simulink model "test_PLC_Drive_Rev3"  (R2020b)
settings: Solver=VariableStepAuto  StartTime=0.0  StopTime=t_stop  RelTol=1e-3
values from neighbouring files (symbols this model uses):
  Controller_sampleTime = 0.001    [PLC_setup_Rev1_02Mar21.m]    (also in PLC_setup_Rev3.m; PLC_setup_Rev4.m)
  Droop_scaling = 0    [PLC_setup_Rev1_02Mar21.m]    (also in PLC_setup_Rev3.m; PLC_setup_Rev4.m)
  VFD_acceleration_model_factor = 0.27*mmul2    (= 0.27)    [PLC_setup_Rev3.m]    (also in PLC_setup_Rev4.m)
  VFD_Adapt_factor_lower_p1458 = 1    [PLC_setup_Rev1_02Mar21.m]    (also in PLC_setup_Rev3.m; PLC_setup_Rev4.m)
  VFD_Adapt_factor_upper_p1459 = 1    [PLC_setup_Rev1_02Mar21.m]    (also in PLC_setup_Rev3.m; PLC_setup_Rev4.m)
  VFD_Curr_limit_var_p0641 = 1    [PLC_setup_Rev1_02Mar21.m]    (also in PLC_setup_Rev3.m; PLC_setup_Rev4.m)
  VFD_Current_limit_p0640 = 430    [PLC_setup_Rev1_02Mar21.m]    (also in PLC_setup_Rev3.m; PLC_setup_Rev4.m)
  VFD_Id_setp_total_r1624 = 73    [PLC_setup_Rev1_02Mar21.m]    (also in PLC_setup_Rev3.m; PLC_setup_Rev4.m)
  VFD_Iq = 1    [PLC_setup_Rev1_02Mar21.m]    (also in PLC_setup_Rev3.m; PLC_setup_Rev4.m)
  VFD_Kp_n_basic_p1460 = 20.174    [PLC_setup_Rev1_02Mar21.m]    (also in PLC_setup_Rev3.m; PLC_setup_Rev4.m)
  VFD_M = inf    [PLC_setup_Rev1_02Mar21.m]    (also in PLC_setup_Rev3.m; PLC_setup_Rev4.m)
  VFD_M_accel_T_smooth_p1517 = 4    [PLC_setup_Rev1_02Mar21.m]    (also in PLC_setup_Rev3.m; PLC_setup_Rev4.m)
  VFD_M_lim_var_fixS_src_p1551 = 1    [PLC_setup_Rev1_02Mar21.m]    (also in PLC_setup_Rev3.m; PLC_setup_Rev4.m)
  VFD_M_max_lower_p1521 = -1345    [PLC_setup_Rev1_02Mar21.m]    (also in PLC_setup_Rev3.m; PLC_setup_Rev4.m)
  VFD_M_max_lower_scal_p1525 = 1    [PLC_setup_Rev1_02Mar21.m]    (also in PLC_setup_Rev3.m; PLC_setup_Rev4.m)
  VFD_M_max_up_mot_scal_p1524 = 1    [PLC_setup_Rev1_02Mar21.m]    (also in PLC_setup_Rev3.m; PLC_setup_Rev4.m)
  VFD_M_max_upper_p1520 = 1345    [PLC_setup_Rev1_02Mar21.m]    (also in PLC_setup_Rev3.m; PLC_setup_Rev4.m)
  VFD_n_act_T_smooth_p1442 = 4    [PLC_setup_Rev1_02Mar21.m]    (also in PLC_setup_Rev3.m; PLC_setup_Rev4.m)
  VFD_n_ctr_Kp_n_up_scal_p1461 = 1    [PLC_setup_Rev1_02Mar21.m]    (also in PLC_setup_Rev3.m; PLC_setup_Rev4.m)
  VFD_n_ctr_Tn_n_up_sca_p1463 = 1    [PLC_setup_Rev1_02Mar21.m]    (also in PLC_setup_Rev3.m; PLC_setup_Rev4.m)
  VFD_n_ctrl_adapt_Kp_lower_p1456 = 0    [PLC_setup_Rev1_02Mar21.m]    (also in PLC_setup_Rev3.m; PLC_setup_Rev4.m)
  VFD_n_ctrl_adapt_Kp_upper_p1457 = 0.1    [PLC_setup_Rev1_02Mar21.m]    (also in PLC_setup_Rev3.m; PLC_setup_Rev4.m)
  VFD_n_ctrl_Adpt_sig_Kp_p1455 = 0    [PLC_setup_Rev1_02Mar21.m]    (also in PLC_setup_Rev3.m; PLC_setup_Rev4.m)
  VFD_n_ctrl_Kp_scal_p1466 = 1    [PLC_setup_Rev1_02Mar21.m]    (also in PLC_setup_Rev3.m; PLC_setup_Rev4.m)
  VFD_n_ctrl_n_lower_p1464 = 0    [PLC_setup_Rev1_02Mar21.m]    (also in PLC_setup_Rev3.m; PLC_setup_Rev4.m)
  VFD_n_ctrl_n_upper_p1465 = 1680    [PLC_setup_Rev1_02Mar21.m]    (also in PLC_setup_Rev3.m; PLC_setup_Rev4.m)
  VFD_n_ctrl_Tn_n_lower_p1462 = 96    [PLC_setup_Rev1_02Mar21.m]    (also in PLC_setup_Rev3.m; PLC_setup_Rev4.m)
  VFD_n_limit_neg_p1086 = -40000    [PLC_setup_Rev1_02Mar21.m]    (also in PLC_setup_Rev3.m; PLC_setup_Rev4.m)
  VFD_n_limit_pos_p1083 = 40000    [PLC_setup_Rev1_02Mar21.m]    (also in PLC_setup_Rev3.m; PLC_setup_Rev4.m)
  VFD_n_limit_setp_p1063 = 40000    [PLC_setup_Rev1_02Mar21.m]    (also in PLC_setup_Rev3.m; PLC_setup_Rev4.m)
  VFD_n_max_p1082 = 1680    [PLC_setup_Rev1_02Mar21.m]    (also in PLC_setup_Rev3.m; PLC_setup_Rev4.m)
  VFD_n_set_filt_1_T_p1416 = 0    [PLC_setup_Rev1_02Mar21.m]    (also in PLC_setup_Rev3.m; PLC_setup_Rev4.m)
  VFD_P_max_gen_p1531 = -375    [PLC_setup_Rev1_02Mar21.m]    (also in PLC_setup_Rev3.m; PLC_setup_Rev4.m)
  VFD_P_max_mot_p1530 = 125    [PLC_setup_Rev1_02Mar21.m]    (also in PLC_setup_Rev3.m; PLC_setup_Rev4.m)
  VFD_PU_I_outp_max_r0289 = 452    [PLC_setup_Rev1_02Mar21.m]    (also in PLC_setup_Rev3.m; PLC_setup_Rev4.m)
  VFD_RFG_ramp_down_time_p1121 = 0.7    [PLC_setup_Rev1_02Mar21.m]    (also in PLC_setup_Rev3.m; PLC_setup_Rev4.m)
  VFD_RFG_ramp_up_time_p1120 = 0.7    [PLC_setup_Rev1_02Mar21.m]    (also in PLC_setup_Rev3.m; PLC_setup_Rev4.m)
  VFD_RFG_t_RD_scal_p1139 = 1    [PLC_setup_Rev1_02Mar21.m]    (also in PLC_setup_Rev3.m; PLC_setup_Rev4.m)
  VFD_RFG_t_RU_scal_p1138 = 1    [PLC_setup_Rev1_02Mar21.m]    (also in PLC_setup_Rev3.m; PLC_setup_Rev4.m)
undefined symbols (not defined in the file or in its folder): DiscIntNeverNeededParam, filt_enc_den, filt_enc_num, filt_NUM, Kp_mul, tau_m, Tn_mul, Tsf
libraries: simulink x49, simulink_extras x1
(part 1 of 2)
settings Model: Creator=Pawel  LastModifiedBy=Pawel

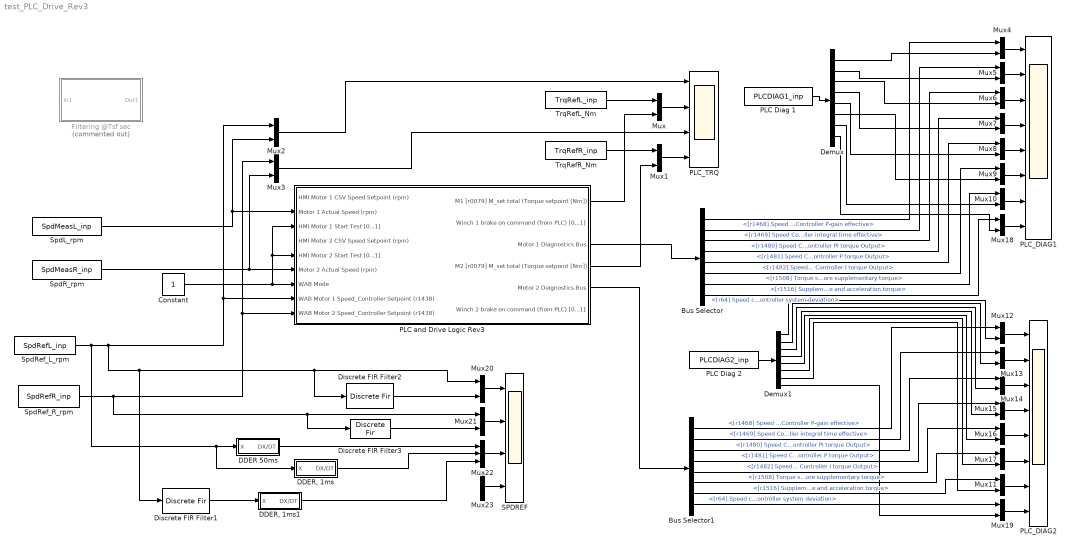
== system test_PLC_Drive_Rev3 ==
  Bus Selector : BusSelector  OutputSignals=signal1.[r1468] Speed Controller P-gain effective,signal1.[r1469] Speed Controller integral time effective,signal1.[r1480] Speed Controller PI torque Output,signal1.[r1481] Speed Controller P torque Output,signal1.[r1482] Speed Controller I torque Output,signal1.[r1508] Torque setpoint before supplementary torque,signal1.[r1516] Supplementary torque and acceleration torque,signal1.[r64] Speed controller system deviation
  Bus Selector1 : BusSelector  OutputSignals=signal1.[r1468] Speed Controller P-gain effective,signal1.[r1469] Speed Controller integral time effective,signal1.[r1480] Speed Controller PI torque Output,signal1.[r1481] Speed Controller P torque Output,signal1.[r1482] Speed Controller I torque Output,signal1.[r1508] Torque setpoint before supplementary torque,signal1.[r1516] Supplementary torque and acceleration torque,signal1.[r64] Speed controller system deviation
  Constant : Constant
  DDER 50ms : Subsystem  TreatAsAtomicUnit=on  SystemSampleTime=0.05
  "DDER, 1ms" : Subsystem  TreatAsAtomicUnit=on  SystemSampleTime=0.001
  "DDER, 1ms1" : Subsystem  TreatAsAtomicUnit=on  SystemSampleTime=0.001
  Demux : Demux  Outputs=8
  Demux1 : Demux  Outputs=8
  Discrete FIR Filter1 : DiscreteFir  Coefficients=filt_NUM  SampleTime=Controller_sampleTime
  Discrete FIR Filter2 : DiscreteFir  Coefficients=filt_NUM  SampleTime=Controller_sampleTime
  Discrete FIR Filter3 : DiscreteFir  Coefficients=filt_NUM  SampleTime=Controller_sampleTime
  Filtering @Tsf sec : Subsystem  Commented=on  TreatAsAtomicUnit=on  SystemSampleTime=Tsf
  Mux{,1..21} (22 alike) : Mux  Inputs=2
  Mux22 : Mux  Inputs=3
  Mux23 : Mux  Inputs=3
  PLC Diag 1 : FromWorkspace  VariableName=PLCDIAG1_inp  OutputAfterFinalValue=Holding final value
  PLC Diag 2 : FromWorkspace  VariableName=PLCDIAG2_inp  OutputAfterFinalValue=Holding final value
  PLC and Drive Logic Rev3 : Subsystem  AncestorBlock=Control_Library_Rev3/PLC and Drive Logic
  PLC_DIAG1 : Scope  NumInputPorts=8
  PLC_DIAG2 : Scope  NumInputPorts=8
  PLC_TRQ : Scope  NumInputPorts=4
  SPDREF : Scope  NumInputPorts=4
  SpdL_rpm : FromWorkspace  VariableName=SpdMeasL_inp  OutputAfterFinalValue=Holding final value
  SpdR_rpm : FromWorkspace  VariableName=SpdMeasR_inp  OutputAfterFinalValue=Holding final value
  SpdRef_L_rpm : FromWorkspace  VariableName=SpdRefL_inp  OutputAfterFinalValue=Holding final value
  SpdRef_R_rpm : FromWorkspace  VariableName=SpdRefR_inp  OutputAfterFinalValue=Holding final value
  TrqRefL_Nm : FromWorkspace  VariableName=TrqRefL_inp  OutputAfterFinalValue=Holding final value
  TrqRefR_Nm : FromWorkspace  VariableName=TrqRefR_inp  OutputAfterFinalValue=Holding final value
  wires:
  Constant/1 -> PLC and Drive Logic Rev3/7(WAB Mode), PLC and Drive Logic Rev3/3(HMI Motor 1 Start Test [0...1]), PLC and Drive Logic Rev3/5(HMI Motor 2 Start Test [0...1])
  PLC and Drive Logic Rev3/1(M1 [r0079] M_set total (Torque setpoint [Nm])) -> Mux/2
  PLC and Drive Logic Rev3/4(M2 [r0079] M_set total (Torque setpoint [Nm])) -> Mux1/2
  Mux/1 -> PLC_TRQ/2
  Mux1/1 -> PLC_TRQ/4
  Mux2/1 -> PLC_TRQ/1
  Mux3/1 -> PLC_TRQ/3
  TrqRefL_Nm/1 -> Mux/1
  TrqRefR_Nm/1 -> Mux1/1
  PLC and Drive Logic Rev3/3(Motor 1 Diagnostics Bus) -> Bus Selector/1
  Mux4/1 -> PLC_DIAG1/1
  Mux6/1 -> PLC_DIAG1/3
  Mux5/1 -> PLC_DIAG1/2
  Mux7/1 -> PLC_DIAG1/4
  Mux9/1 -> PLC_DIAG1/6
  Mux8/1 -> PLC_DIAG1/5
  Mux10/1 -> PLC_DIAG1/7
  Bus Selector/1 -> Mux4/1  "<[r1468] Speed Controller P-gain effective>"
  Bus Selector/2 -> Mux5/1  "<[r1469] Speed Controller integral time effective>"
  Bus Selector/3 -> Mux6/1  "<[r1480] Speed Controller PI torque Output>"
  Bus Selector/4 -> Mux7/1  "<[r1481] Speed Controller P torque Output>"
  Bus Selector/5 -> Mux8/1  "<[r1482] Speed Controller I torque Output>"
  Bus Selector/6 -> Mux9/1  "<[r1508] Torque setpoint before supplementary torque>"
  Bus Selector/7 -> Mux10/1  "<[r1516] Supplementary torque and acceleration torque>"
  PLC and Drive Logic Rev3/5(Motor 2 Diagnostics Bus) -> Bus Selector1/1
  Bus Selector1/7 -> Mux11/1  "<[r1516] Supplementary torque and acceleration torque>"
  Bus Selector1/6 -> Mux17/1  "<[r1508] Torque setpoint before supplementary torque>"
  Bus Selector1/5 -> Mux16/1  "<[r1482] Speed Controller I torque Output>"
  Bus Selector1/4 -> Mux15/1  "<[r1481] Speed Controller P torque Output>"
  Bus Selector1/3 -> Mux14/1  "<[r1480] Speed Controller PI torque Output>"
  Bus Selector1/2 -> Mux13/1  "<[r1469] Speed Controller integral time effective>"
  Bus Selector1/1 -> Mux12/1  "<[r1468] Speed Controller P-gain effective>"
  Mux11/1 -> PLC_DIAG2/7
  Mux16/1 -> PLC_DIAG2/5
  Mux17/1 -> PLC_DIAG2/6
  Mux15/1 -> PLC_DIAG2/4
  Mux13/1 -> PLC_DIAG2/2
  Mux14/1 -> PLC_DIAG2/3
  Mux12/1 -> PLC_DIAG2/1
  SpdRef_R_rpm/1 -> PLC and Drive Logic Rev3/9(WAB Motor 2 Speed_Controller Setpoint (r1438)), Mux3/1, Discrete FIR Filter3/1, Mux21/1
  SpdRef_L_rpm/1 -> "DDER, 1ms"/1(X), DDER 50ms/1(X), PLC and Drive Logic Rev3/8(WAB Motor 1 Speed_Controller Setpoint (r1438)), Mux2/1, Discrete FIR Filter1/1, Discrete FIR Filter2/1, Mux20/1
  SpdR_rpm/1 -> PLC and Drive Logic Rev3/6(Motor 2 Actual Speed (rpm)), Mux3/2
  SpdL_rpm/1 -> PLC and Drive Logic Rev3/2(Motor 1 Actual Speed (rpm)), Mux2/2
  PLC Diag 1/1 -> Demux/1
  Demux/1 -> Mux4/2
  Demux/2 -> Mux5/2
  Demux/3 -> Mux6/2
  Demux/4 -> Mux7/2
  Demux/5 -> Mux8/2
  Demux/6 -> Mux9/2
  Demux/7 -> Mux10/2
  PLC Diag 2/1 -> Demux1/1
  Demux1/1 -> Mux12/2
  Demux1/2 -> Mux13/2
  Demux1/3 -> Mux14/2
  Demux1/4 -> Mux15/2
  Demux1/5 -> Mux16/2
  Demux1/6 -> Mux17/2
  Demux1/7 -> Mux11/2
  Mux18/1 -> PLC_DIAG1/8
  Mux19/1 -> PLC_DIAG2/8
  Bus Selector/8 -> Mux18/1  "<[r64] Speed controller system deviation>"
  Bus Selector1/8 -> Mux19/1  "<[r64] Speed controller system deviation>"
  Demux/8 -> Mux18/2
  Demux1/8 -> Mux19/2
  Mux20/1 -> SPDREF/1
  Mux21/1 -> SPDREF/2
  Mux23/1 -> SPDREF/4
  Mux22/1 -> SPDREF/3
  DDER 50ms/1(DX/DT) -> Mux22/1
  "DDER, 1ms"/1(DX/DT) -> Mux22/2
  "DDER, 1ms1"/1(DX/DT) -> Mux22/3
  Discrete FIR Filter1/1 -> "DDER, 1ms1"/1(X)
  Discrete FIR Filter2/1 -> Mux20/2
  Discrete FIR Filter3/1 -> Mux21/2

== system test_PLC_Drive_Rev3/DDER 50ms ==
  X : Inport
  Discrete Derivative : simulink/Discrete/Discrete Derivative  gainval=1.0  ICPrevScaledInput=0.0  OutMin=[]  OutMax=[]  OutDataType=fixdt(1, 16)  OutScaling=2^-10  DoSatur=off
  DX/DT : Outport
  wires:
  Discrete Derivative/1 -> DX/DT/1
  X/1 -> Discrete Derivative/1

== system test_PLC_Drive_Rev3/DDER, 1ms ==
  X : Inport
  Discrete Derivative : simulink/Discrete/Discrete Derivative  gainval=1.0  ICPrevScaledInput=0.0  OutMin=[]  OutMax=[]  OutDataType=fixdt(1, 16)  OutScaling=2^-10  DoSatur=off
  DX/DT : Outport
  wires:
  X/1 -> Discrete Derivative/1
  Discrete Derivative/1 -> DX/DT/1

== system test_PLC_Drive_Rev3/DDER, 1ms1 ==
  X : Inport
  Discrete Derivative : simulink/Discrete/Discrete Derivative  gainval=1.0  ICPrevScaledInput=0.0  OutMin=[]  OutMax=[]  OutDataType=fixdt(1, 16)  OutScaling=2^-10  DoSatur=off
  DX/DT : Outport
  wires:
  Discrete Derivative/1 -> DX/DT/1
  X/1 -> Discrete Derivative/1

== system test_PLC_Drive_Rev3/Filtering @Tsf sec ==
  In1 : Inport
  Filter2 : simulink_extras/Additional Discrete/Discrete Transfer Fcn (with initial outputs)  N=filt_enc_num  D=filt_enc_den  U0=qA_0  Y0=qA_0  TS=-1
      settings: SourceProductBaseCode=SL
  Out1 : Outport

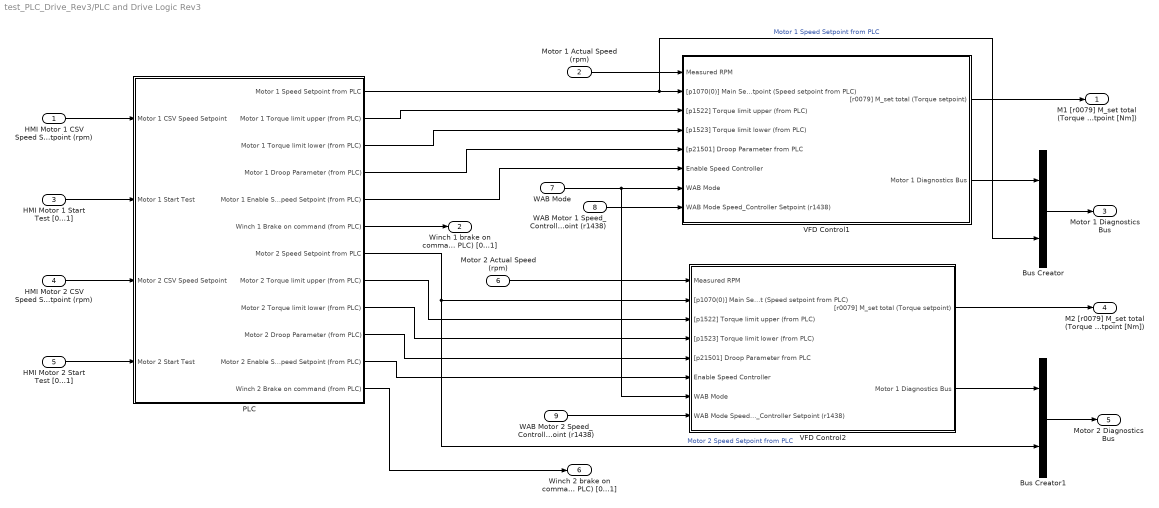
== system test_PLC_Drive_Rev3/PLC and Drive Logic Rev3 ==
  HMI Motor 1 CSV Speed Setpoint (rpm) : Inport
  Motor 1 Actual Speed (rpm) : Inport  Port=2
  HMI Motor 1 Start Test [0...1] : Inport  Port=3
  HMI Motor 2 CSV Speed Setpoint (rpm) : Inport  Port=4
  HMI Motor 2 Start Test [0...1] : Inport  Port=5
  Motor 2 Actual Speed (rpm) : Inport  Port=6
  WAB Mode : Inport  Port=7
  WAB Motor 1 Speed_Controller Setpoint (r1438) : Inport  Port=8
  WAB Motor 2 Speed_Controller Setpoint (r1438) : Inport  Port=9
  Bus Creator : BusCreator  Inputs=2
  Bus Creator1 : BusCreator  Inputs=2
  PLC : Subsystem  TreatAsAtomicUnit=on  SystemSampleTime=Controller_sampleTime
  VFD Control1 : Subsystem  AncestorBlock=Control_Library_Rev3/VFD Control  TreatAsAtomicUnit=on  SystemSampleTime=Controller_sampleTime
  VFD Control2 : Subsystem  AncestorBlock=Control_Library_Rev3/VFD Control  TreatAsAtomicUnit=on  SystemSampleTime=Controller_sampleTime
  M1 [r0079] M_set total (Torque setpoint [Nm]) : Outport
  Winch 1 brake on command (from PLC) [0...1] : Outport  Port=2
  Motor 1 Diagnostics Bus : Outport  Port=3
  M2 [r0079] M_set total (Torque setpoint [Nm]) : Outport  Port=4
  Motor 2 Diagnostics Bus : Outport  Port=5
  Winch 2 brake on command (from PLC) [0...1] : Outport  Port=6
  wires:
  PLC/3(Motor 1 Torque limit lower (from PLC)) -> VFD Control1/4("[p1523] Torque limit lower (from PLC)")
  Motor 1 Actual Speed (rpm)/1 -> VFD Control1/1(Measured RPM)
  PLC/2(Motor 1 Torque limit upper (from PLC)) -> VFD Control1/3("[p1522] Torque limit upper (from PLC)")
  PLC/1(Motor 1 Speed Setpoint from PLC) -> VFD Control1/2("[p1070(0)] Main Setpoint (Speed setpoint from PLC)"), Bus Creator/2  "Motor 1 Speed Setpoint from PLC"
  HMI Motor 1 Start Test [0...1]/1 -> PLC/2(Motor 1 Start Test)
  VFD Control1/1("[r0079] M_set total (Torque setpoint)") -> M1 [r0079] M_set total (Torque setpoint [Nm])/1
  HMI Motor 1 CSV Speed Setpoint (rpm)/1 -> PLC/1(Motor 1 CSV Speed Setpoint)
  PLC/4(Motor 1 Droop Parameter (from PLC)) -> VFD Control1/5("[p21501] Droop Parameter from PLC")
  PLC/5(Motor 1 Enable Speed Setpoint (from PLC)) -> VFD Control1/6(Enable Speed Controller)
  VFD Control1/2(Motor 1 Diagnostics Bus) -> Bus Creator/1
  Bus Creator/1 -> Motor 1 Diagnostics Bus/1
  Bus Creator1/1 -> Motor 2 Diagnostics Bus/1
  VFD Control2/2(Motor 1 Diagnostics Bus) -> Bus Creator1/1
  VFD Control2/1("[r0079] M_set total (Torque setpoint)") -> M2 [r0079] M_set total (Torque setpoint [Nm])/1
  PLC/6(Winch 1 Brake on command (from PLC)) -> Winch 1 brake on command (from PLC) [0...1]/1
  HMI Motor 2 CSV Speed Setpoint (rpm)/1 -> PLC/3(Motor 2 CSV Speed Setpoint)
  HMI Motor 2 Start Test [0...1]/1 -> PLC/4(Motor 2 Start Test)
  Motor 2 Actual Speed (rpm)/1 -> VFD Control2/1(Measured RPM)
  PLC/7(Motor 2 Speed Setpoint from PLC) -> Bus Creator1/2, VFD Control2/2("[p1070(0)] Main Setpoint (Speed setpoint from PLC)")  "Motor 2 Speed Setpoint from PLC"
  PLC/8(Motor 2 Torque limit upper (from PLC)) -> VFD Control2/3("[p1522] Torque limit upper (from PLC)")
  PLC/9(Motor 2 Torque limit lower (from PLC)) -> VFD Control2/4("[p1523] Torque limit lower (from PLC)")
  PLC/10(Motor 2 Droop Parameter (from PLC)) -> VFD Control2/5("[p21501] Droop Parameter from PLC")
  PLC/11(Motor 2 Enable Speed Setpoint (from PLC)) -> VFD Control2/6(Enable Speed Controller)
  PLC/12(Winch 2 Brake on command (from PLC)) -> Winch 2 brake on command (from PLC) [0...1]/1
  WAB Motor 1 Speed_Controller Setpoint (r1438)/1 -> VFD Control1/8(WAB Mode Speed_Controller Setpoint (r1438))
  WAB Mode/1 -> VFD Control2/7(WAB Mode), VFD Control1/7(WAB Mode)
  WAB Motor 2 Speed_Controller Setpoint (r1438)/1 -> VFD Control2/8(WAB Mode Speed_Controller Setpoint (r1438))

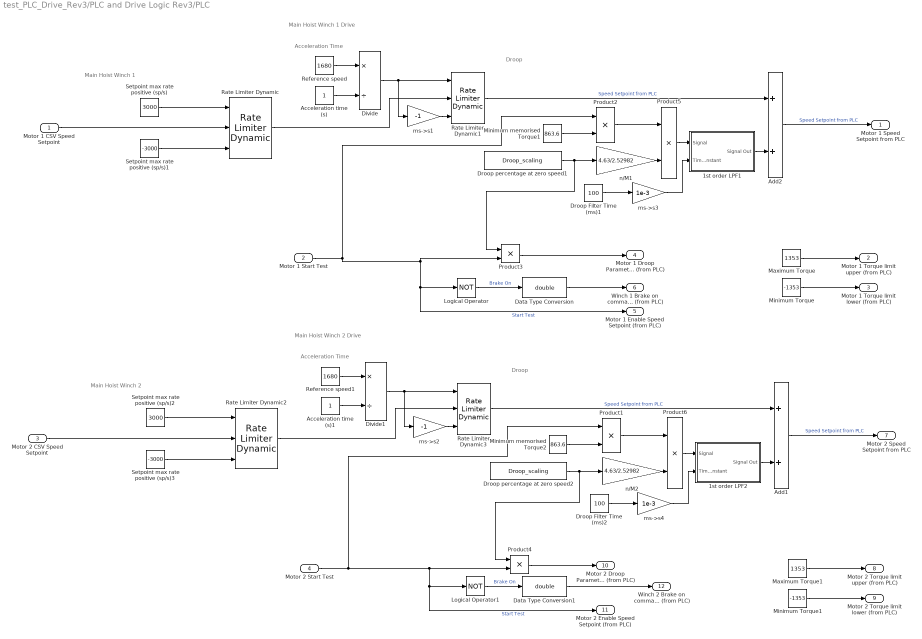
== system test_PLC_Drive_Rev3/PLC and Drive Logic Rev3/PLC ==
  note: Main Hoist Winch 1 Drive
  note: Acceleration Time
  note: Droop
  note: Main Hoist Winch 1
  note: Main Hoist Winch 2 Drive
  note: Acceleration Time
  note: Droop
  note: Main Hoist Winch 2
  Motor 1 CSV Speed Setpoint : Inport
  Motor 1 Start Test : Inport  Port=2
  Motor 2 CSV Speed Setpoint : Inport  Port=3
  Motor 2 Start Test : Inport  Port=4
  1st order LPF1 : Subsystem  mask{time_constant=0.1, Yo=0}
      mask prompts: time_constant "Time Constant (s)"; Yo "Initial Condition"
  1st order LPF2 : Subsystem  mask{time_constant=0.1, Yo=0}
      mask prompts: time_constant "Time Constant (s)"; Yo "Initial Condition"
  Acceleration time (s) : Constant
  Acceleration time (s)1 : Constant
  Add1 : Sum
  Add2 : Sum
  Data Type Conversion : DataTypeConversion  OutDataTypeStr=double
  Data Type Conversion1 : DataTypeConversion  OutDataTypeStr=double
  Divide : Product  Inputs=*/
  Divide1 : Product  Inputs=*/
  Droop Filter Time (ms)1 : Constant  Value=100
  Droop Filter Time (ms)2 : Constant  Value=100
  Droop percentage at zero speed1 : Constant  Value=Droop_scaling
  Droop percentage at zero speed2 : Constant  Value=Droop_scaling
  Logical Operator : Logic  Operator=NOT  AllPortsSameDT=off  OutDataTypeStr=boolean
  Logical Operator1 : Logic  Operator=NOT  AllPortsSameDT=off  OutDataTypeStr=boolean
  Maximum Torque : Constant  Value=1353
  Maximum Torque1 : Constant  Value=1353
  Minimum Torque : Constant  Value=-1353
  Minimum Torque1 : Constant  Value=-1353
  Minimum memorised Torque1 : Constant  Value=863.6
  Minimum memorised Torque2 : Constant  Value=863.6
  Product{1..2,5..6} (4 alike) : Product  Inputs=**
  Product3 : Product
  Product4 : Product
  Rate Limiter Dynamic{,1..3} (4 alike) : simulink/Discontinuities/Rate Limiter Dynamic
  Reference speed : Constant  Value=1680
  Reference speed1 : Constant  Value=1680
  Setpoint max rate positive (sp/s) : Constant  Value=3000
  Setpoint max rate positive (sp/s)1 : Constant  Value=-3000
  Setpoint max rate positive (sp/s)2 : Constant  Value=3000
  Setpoint max rate positive (sp/s)3 : Constant  Value=-3000
  ms->s1 : Gain  Gain=-1
  ms->s2 : Gain  Gain=-1
  ms->s3 : Gain  Gain=1e-3
  ms->s4 : Gain  Gain=1e-3
  n/M1 : Gain  Gain=4.63/2.52982
  n/M2 : Gain  Gain=4.63/2.52982
  Motor 1 Speed Setpoint from PLC : Outport
  Motor 1 Torque limit upper (from PLC) : Outport  Port=2
  Motor 1 Torque limit lower (from PLC) : Outport  Port=3
  Motor 1 Droop Parameter (from PLC) : Outport  Port=4
  Motor 1 Enable Speed Setpoint (from PLC) : Outport  Port=5
  Winch 1 Brake on command (from PLC) : Outport  Port=6
  Motor 2 Speed Setpoint from PLC : Outport  Port=7
  Motor 2 Torque limit upper (from PLC) : Outport  Port=8
  Motor 2 Torque limit lower (from PLC) : Outport  Port=9
  Motor 2 Droop Parameter (from PLC) : Outport  Port=10
  Motor 2 Enable Speed Setpoint (from PLC) : Outport  Port=11
  Winch 2 Brake on command (from PLC) : Outport  Port=12
  wires:
  Product2/1 -> Product5/1
  n/M1/1 -> Product5/2
  ms->s1/1 -> Rate Limiter Dynamic1/3
  ms->s3/1 -> 1st order LPF1/2(Time Constant)
  Divide/1 -> ms->s1/1, Rate Limiter Dynamic1/1
  Setpoint max rate positive (sp/s)/1 -> Rate Limiter Dynamic/1
  Setpoint max rate positive (sp/s)1/1 -> Rate Limiter Dynamic/3
  Product5/1 -> 1st order LPF1/1(Signal)
  Droop Filter Time (ms)1/1 -> ms->s3/1
  1st order LPF1/1(Signal Out) -> Add2/2
  Droop percentage at zero speed1/1 -> Product3/1, n/M1/1
  Rate Limiter Dynamic/1 -> Rate Limiter Dynamic1/2
  Minimum memorised Torque1/1 -> Product2/2
  Reference speed/1 -> Divide/1
  Acceleration time (s)/1 -> Divide/2
  Add2/1 -> Motor 1 Speed Setpoint from PLC/1  "Speed Setpoint from PLC"
  Maximum Torque/1 -> Motor 1 Torque limit upper (from PLC)/1
  Minimum Torque/1 -> Motor 1 Torque limit lower (from PLC)/1
  Rate Limiter Dynamic1/1 -> Add2/1  "Speed Setpoint from PLC"
  Motor 1 Start Test/1 -> Motor 1 Enable Speed Setpoint (from PLC)/1, Logical Operator/1, Product3/2, Product2/1  "Start Test"
  Product3/1 -> Motor 1 Droop Parameter (from PLC)/1
  Logical Operator/1 -> Data Type Conversion/1  "Brake On"
  Data Type Conversion/1 -> Winch 1 Brake on command (from PLC)/1
  Motor 1 CSV Speed Setpoint/1 -> Rate Limiter Dynamic/2
  Motor 2 CSV Speed Setpoint/1 -> Rate Limiter Dynamic2/2
  Data Type Conversion1/1 -> Winch 2 Brake on command (from PLC)/1
  Logical Operator1/1 -> Data Type Conversion1/1  "Brake On"
  Product4/1 -> Motor 2 Droop Parameter (from PLC)/1
  Motor 2 Start Test/1 -> Product1/1, Motor 2 Enable Speed Setpoint (from PLC)/1, Logical Operator1/1, Product4/2  "Start Test"
  Rate Limiter Dynamic3/1 -> Add1/1  "Speed Setpoint from PLC"
  Minimum Torque1/1 -> Motor 2 Torque limit lower (from PLC)/1
  Maximum Torque1/1 -> Motor 2 Torque limit upper (from PLC)/1
  Add1/1 -> Motor 2 Speed Setpoint from PLC/1  "Speed Setpoint from PLC"
  Acceleration time (s)1/1 -> Divide1/2
  Reference speed1/1 -> Divide1/1
  Minimum memorised Torque2/1 -> Product1/2
  Rate Limiter Dynamic2/1 -> Rate Limiter Dynamic3/2
  Droop percentage at zero speed2/1 -> n/M2/1, Product4/1
  1st order LPF2/1(Signal Out) -> Add1/2
  Droop Filter Time (ms)2/1 -> ms->s4/1
  Product6/1 -> 1st order LPF2/1(Signal)
  Setpoint max rate positive (sp/s)3/1 -> Rate Limiter Dynamic2/3
  Setpoint max rate positive (sp/s)2/1 -> Rate Limiter Dynamic2/1
  Divide1/1 -> Rate Limiter Dynamic3/1, ms->s2/1
  ms->s4/1 -> 1st order LPF2/2(Time Constant)
  ms->s2/1 -> Rate Limiter Dynamic3/3
  n/M2/1 -> Product6/2
  Product1/1 -> Product6/1

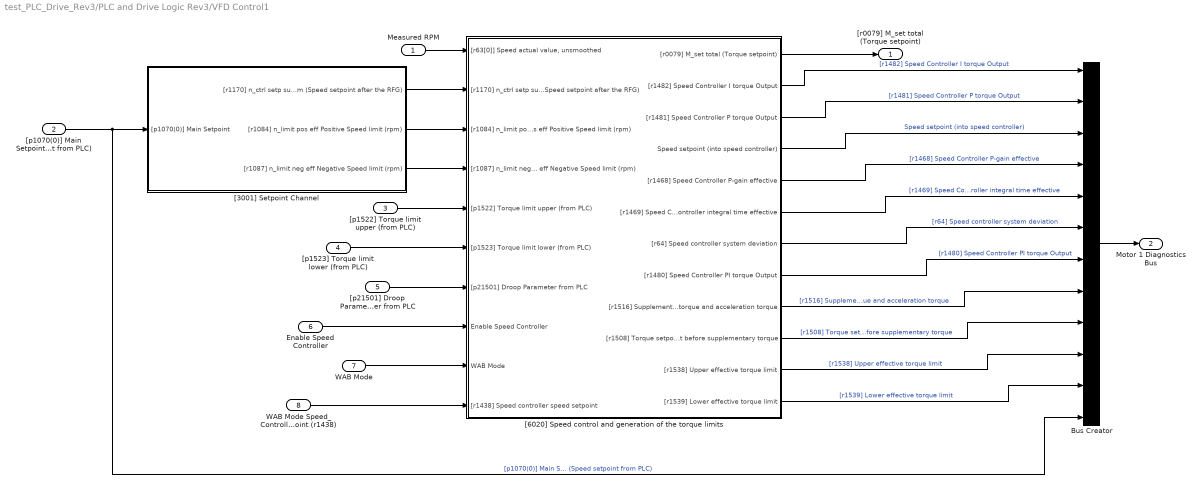
== system test_PLC_Drive_Rev3/PLC and Drive Logic Rev3/VFD Control1 ==
  Measured RPM : Inport
  "[p1070(0)] Main Setpoint (Speed setpoint from PLC)" : Inport  Port=2
  "[p1522] Torque limit upper (from PLC)" : Inport  Port=3
  "[p1523] Torque limit lower (from PLC)" : Inport  Port=4
  "[p21501] Droop Parameter from PLC" : Inport  Port=5
  Enable Speed Controller : Inport  Port=6
  WAB Mode : Inport  Port=7
  WAB Mode Speed_Controller Setpoint (r1438) : Inport  Port=8
  Bus Creator : BusCreator  Inputs=12
  "[3001] Setpoint Channel " : Subsystem
  "[6020] Speed control and generation of the torque limits " : Subsystem
  "[r0079] M_set total (Torque setpoint)" : Outport  VectorParamsAs1DForOutWhenUnconnected=off
  Motor 1 Diagnostics Bus : Outport  Port=2
  wires:
  "[6020] Speed control and generation of the torque limits "/12("[r1539] Lower effective torque limit") -> Bus Creator/11  "[r1539] Lower effective torque limit"
  "[6020] Speed control and generation of the torque limits "/11("[r1538] Upper effective torque limit") -> Bus Creator/10  "[r1538] Upper effective torque limit"
  "[6020] Speed control and generation of the torque limits "/10("[r1508] Torque setpoint before supplementary torque") -> Bus Creator/9  "[r1508] Torque setpoint before supplementary torque"
  "[6020] Speed control and generation of the torque limits "/9("[r1516] Supplementary torque and acceleration torque ") -> Bus Creator/8  "[r1516] Supplementary torque and acceleration torque"
  "[6020] Speed control and generation of the torque limits "/8("[r1480] Speed Controller PI torque Output") -> Bus Creator/7  "[r1480] Speed Controller PI torque Output"
  "[6020] Speed control and generation of the torque limits "/7("[r64] Speed controller system deviation") -> Bus Creator/6  "[r64] Speed controller system deviation"
  "[6020] Speed control and generation of the torque limits "/6("[r1469] Speed Controller integral time effective") -> Bus Creator/5  "[r1469] Speed Controller integral time effective"
  "[6020] Speed control and generation of the torque limits "/5("[r1468] Speed Controller P-gain effective") -> Bus Creator/4  "[r1468] Speed Controller P-gain effective"
  Bus Creator/1 -> Motor 1 Diagnostics Bus/1
  WAB Mode Speed_Controller Setpoint (r1438)/1 -> "[6020] Speed control and generation of the torque limits "/10("[r1438] Speed controller speed setpoint")
  WAB Mode/1 -> "[6020] Speed control and generation of the torque limits "/9(WAB Mode)
  "[6020] Speed control and generation of the torque limits "/2("[r1482] Speed Controller I torque Output") -> Bus Creator/1  "[r1482] Speed Controller I torque Output"
  "[6020] Speed control and generation of the torque limits "/3("[r1481] Speed Controller P torque Output") -> Bus Creator/2  "[r1481] Speed Controller P torque Output"
  Measured RPM/1 -> "[6020] Speed control and generation of the torque limits "/1("[r63[0]] Speed actual value, unsmoothed")
  "[p1070(0)] Main Setpoint (Speed setpoint from PLC)"/1 -> Bus Creator/12, "[3001] Setpoint Channel "/1("[p1070(0)] Main Setpoint")  "[p1070(0)] Main Setpoint (Speed setpoint from PLC)"
  "[3001] Setpoint Channel "/1("[r1170] n_ctrl setp sum (Speed setpoint after the RFG)") -> "[6020] Speed control and generation of the torque limits "/2("[r1170] n_ctrl setp sum (Speed setpoint after the RFG)")
  "[3001] Setpoint Channel "/2("[r1084] n_limit pos eff Positive Speed limit (rpm)") -> "[6020] Speed control and generation of the torque limits "/3("[r1084] n_limit pos eff Positive Speed limit (rpm)")
  "[3001] Setpoint Channel "/3("[r1087] n_limit neg eff Negative Speed limit (rpm)") -> "[6020] Speed control and generation of the torque limits "/4("[r1087] n_limit neg eff Negative Speed limit (rpm)")
  "[6020] Speed control and generation of the torque limits "/4(Speed setpoint (into speed controller)) -> Bus Creator/3  "Speed setpoint (into speed controller)"
  "[6020] Speed control and generation of the torque limits "/1("[r0079] M_set total (Torque setpoint)") -> "[r0079] M_set total (Torque setpoint)"/1
  "[p1523] Torque limit lower (from PLC)"/1 -> "[6020] Speed control and generation of the torque limits "/6("[p1523] Torque limit lower (from PLC)")
  "[p1522] Torque limit upper (from PLC)"/1 -> "[6020] Speed control and generation of the torque limits "/5("[p1522] Torque limit upper (from PLC)")
  "[p21501] Droop Parameter from PLC"/1 -> "[6020] Speed control and generation of the torque limits "/7("[p21501] Droop Parameter from PLC")
  Enable Speed Controller/1 -> "[6020] Speed control and generation of the torque limits "/8(Enable Speed Controller)

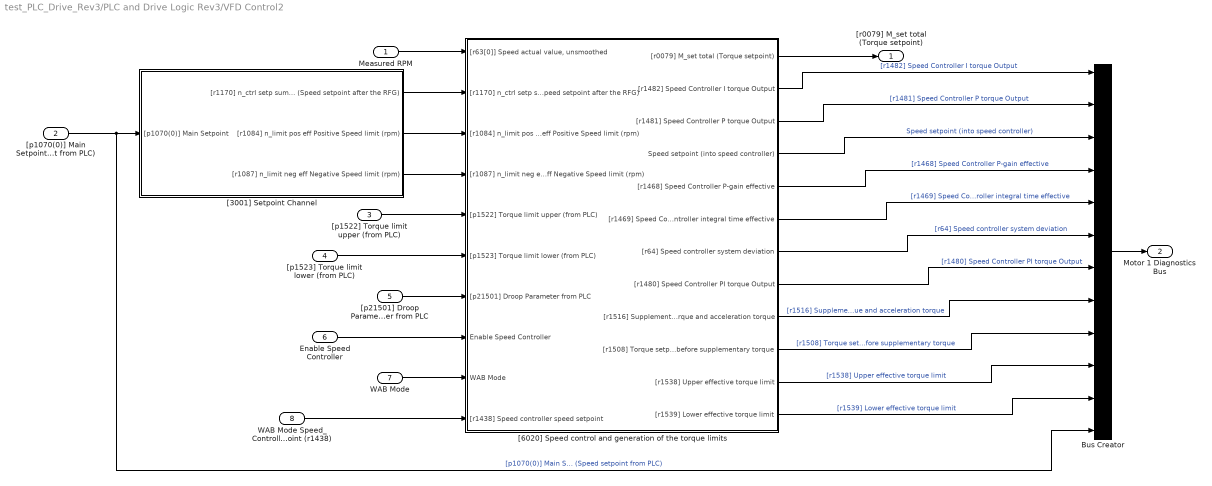
== system test_PLC_Drive_Rev3/PLC and Drive Logic Rev3/VFD Control2 ==
  Measured RPM : Inport
  "[p1070(0)] Main Setpoint (Speed setpoint from PLC)" : Inport  Port=2
  "[p1522] Torque limit upper (from PLC)" : Inport  Port=3
  "[p1523] Torque limit lower (from PLC)" : Inport  Port=4
  "[p21501] Droop Parameter from PLC" : Inport  Port=5
  Enable Speed Controller : Inport  Port=6
  WAB Mode : Inport  Port=7
  WAB Mode Speed_Controller Setpoint (r1438) : Inport  Port=8
  Bus Creator : BusCreator  Inputs=12
  "[3001] Setpoint Channel " : Subsystem
  "[6020] Speed control and generation of the torque limits " : Subsystem
  "[r0079] M_set total (Torque setpoint)" : Outport  VectorParamsAs1DForOutWhenUnconnected=off
  Motor 1 Diagnostics Bus : Outport  Port=2
  wires:
  "[6020] Speed control and generation of the torque limits "/12("[r1539] Lower effective torque limit") -> Bus Creator/11  "[r1539] Lower effective torque limit"
  "[6020] Speed control and generation of the torque limits "/11("[r1538] Upper effective torque limit") -> Bus Creator/10  "[r1538] Upper effective torque limit"
  "[6020] Speed control and generation of the torque limits "/10("[r1508] Torque setpoint before supplementary torque") -> Bus Creator/9  "[r1508] Torque setpoint before supplementary torque"
  "[6020] Speed control and generation of the torque limits "/9("[r1516] Supplementary torque and acceleration torque ") -> Bus Creator/8  "[r1516] Supplementary torque and acceleration torque"
  "[6020] Speed control and generation of the torque limits "/8("[r1480] Speed Controller PI torque Output") -> Bus Creator/7  "[r1480] Speed Controller PI torque Output"
  "[6020] Speed control and generation of the torque limits "/7("[r64] Speed controller system deviation") -> Bus Creator/6  "[r64] Speed controller system deviation"
  "[6020] Speed control and generation of the torque limits "/6("[r1469] Speed Controller integral time effective") -> Bus Creator/5  "[r1469] Speed Controller integral time effective"
  "[6020] Speed control and generation of the torque limits "/5("[r1468] Speed Controller P-gain effective") -> Bus Creator/4  "[r1468] Speed Controller P-gain effective"
  Bus Creator/1 -> Motor 1 Diagnostics Bus/1
  WAB Mode Speed_Controller Setpoint (r1438)/1 -> "[6020] Speed control and generation of the torque limits "/10("[r1438] Speed controller speed setpoint")
  WAB Mode/1 -> "[6020] Speed control and generation of the torque limits "/9(WAB Mode)
  "[6020] Speed control and generation of the torque limits "/2("[r1482] Speed Controller I torque Output") -> Bus Creator/1  "[r1482] Speed Controller I torque Output"
  "[6020] Speed control and generation of the torque limits "/3("[r1481] Speed Controller P torque Output") -> Bus Creator/2  "[r1481] Speed Controller P torque Output"
  Measured RPM/1 -> "[6020] Speed control and generation of the torque limits "/1("[r63[0]] Speed actual value, unsmoothed")
  "[p1070(0)] Main Setpoint (Speed setpoint from PLC)"/1 -> Bus Creator/12, "[3001] Setpoint Channel "/1("[p1070(0)] Main Setpoint")  "[p1070(0)] Main Setpoint (Speed setpoint from PLC)"
  "[3001] Setpoint Channel "/1("[r1170] n_ctrl setp sum (Speed setpoint after the RFG)") -> "[6020] Speed control and generation of the torque limits "/2("[r1170] n_ctrl setp sum (Speed setpoint after the RFG)")
  "[3001] Setpoint Channel "/2("[r1084] n_limit pos eff Positive Speed limit (rpm)") -> "[6020] Speed control and generation of the torque limits "/3("[r1084] n_limit pos eff Positive Speed limit (rpm)")
  "[3001] Setpoint Channel "/3("[r1087] n_limit neg eff Negative Speed limit (rpm)") -> "[6020] Speed control and generation of the torque limits "/4("[r1087] n_limit neg eff Negative Speed limit (rpm)")
  "[6020] Speed control and generation of the torque limits "/4(Speed setpoint (into speed controller)) -> Bus Creator/3  "Speed setpoint (into speed controller)"
  "[6020] Speed control and generation of the torque limits "/1("[r0079] M_set total (Torque setpoint)") -> "[r0079] M_set total (Torque setpoint)"/1
  "[p1523] Torque limit lower (from PLC)"/1 -> "[6020] Speed control and generation of the torque limits "/6("[p1523] Torque limit lower (from PLC)")
  "[p1522] Torque limit upper (from PLC)"/1 -> "[6020] Speed control and generation of the torque limits "/5("[p1522] Torque limit upper (from PLC)")
  "[p21501] Droop Parameter from PLC"/1 -> "[6020] Speed control and generation of the torque limits "/7("[p21501] Droop Parameter from PLC")
  Enable Speed Controller/1 -> "[6020] Speed control and generation of the torque limits "/8(Enable Speed Controller)

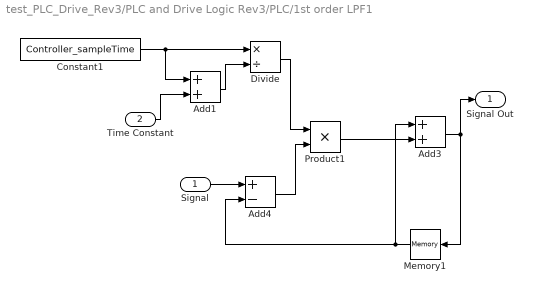
== system test_PLC_Drive_Rev3/PLC and Drive Logic Rev3/PLC/1st order LPF1 ==
  Signal : Inport
  Time Constant : Inport  Port=2
  Add1 : Sum
  Add3 : Sum
  Add4 : Sum  Inputs=+-
  Constant1 : Constant  Value=Controller_sampleTime
  Divide : Product  Inputs=*/
  Memory1 : Memory  InitialCondition=Yo  InheritSampleTime=on
  Product1 : Product  RndMeth=Zero
  Signal Out : Outport  VectorParamsAs1DForOutWhenUnconnected=off
  wires:
  Add1/1 -> Divide/2
  Divide/1 -> Product1/1
  Add3/1 -> Memory1/1, Signal Out/1
  Product1/1 -> Add3/2
  Memory1/1 -> Add4/2, Add3/1
  Add4/1 -> Product1/2
  Time Constant/1 -> Add1/2
  Constant1/1 -> Add1/1, Divide/1
  Signal/1 -> Add4/1

== system test_PLC_Drive_Rev3/PLC and Drive Logic Rev3/PLC/1st order LPF2 ==
  Signal : Inport
  Time Constant : Inport  Port=2
  Add1 : Sum
  Add3 : Sum
  Add4 : Sum  Inputs=+-
  Constant1 : Constant  Value=Controller_sampleTime
  Divide : Product  Inputs=*/
  Memory1 : Memory  InitialCondition=Yo  InheritSampleTime=on
  Product1 : Product  RndMeth=Zero
  Signal Out : Outport  VectorParamsAs1DForOutWhenUnconnected=off
  wires:
  Signal/1 -> Add4/1
  Constant1/1 -> Divide/1, Add1/1
  Time Constant/1 -> Add1/2
  Add4/1 -> Product1/2
  Memory1/1 -> Add3/1, Add4/2
  Product1/1 -> Add3/2
  Add3/1 -> Signal Out/1, Memory1/1
  Divide/1 -> Product1/1
  Add1/1 -> Divide/2

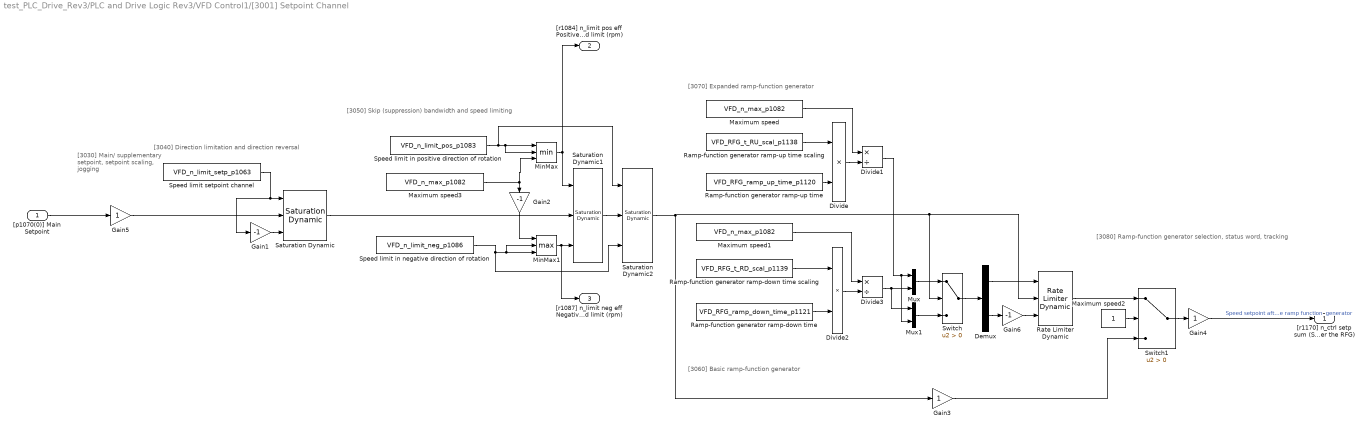
== system test_PLC_Drive_Rev3/PLC and Drive Logic Rev3/VFD Control1/[3001] Setpoint Channel  ==
  note: [3080] Ramp-function generator selection,
      | status word, tracking
  note: [3070] Expanded ramp-function generator
  note: [3040] Direction limitation and direction reversal
  note: [3050] Skip (suppression) bandwidth
      |  and speed limiting
  note: [3060] Basic ramp-function generator
  note: [3030] Main/
      | supplementary
      | setpoint,
      | setpoint
      | scaling,
      | jogging
  "[p1070(0)] Main Setpoint" : Inport
  Demux : Demux  Outputs=2
  Divide : Product  Inputs=**
  Divide1 : Product  Inputs=*/
  Divide2 : Product  Inputs=**
  Divide3 : Product  Inputs=*/
  Gain1 : Gain  Gain=-1
  Gain2 : Gain  Gain=-1
  Gain3 : Gain
  Gain4 : Gain
  Gain5 : Gain
  Gain6 : Gain  Gain=-1
  Maximum speed : Constant  Value=VFD_n_max_p1082
  Maximum speed1 : Constant  Value=VFD_n_max_p1082
  Maximum speed2 : Constant
  Maximum speed3 : Constant  Value=VFD_n_max_p1082
  MinMax : MinMax  Inputs=3
  MinMax1 : MinMax  Function=max  Inputs=3
  Mux : Mux  Inputs=2
  Mux1 : Mux  Inputs=2
  Ramp-function generator ramp-down time : Constant  Value=VFD_RFG_ramp_down_time_p1121
  Ramp-function generator ramp-down time scaling : Constant  Value=VFD_RFG_t_RD_scal_p1139  VectorParams1D=off
  "Ramp-function generator ramp-up time " : Constant  Value=VFD_RFG_ramp_up_time_p1120
  "Ramp-function generator ramp-up time scaling " : Constant  Value=VFD_RFG_t_RU_scal_p1138
  Rate Limiter Dynamic : simulink/Discontinuities/Rate Limiter Dynamic
  Saturation Dynamic : simulink/Discontinuities/Saturation Dynamic  OutMin=[]  OutMax=[]  OutDataTypeStr=Inherit: Same as second input  OutDataType=fixdt(1, 16)  OutScaling=2^-10  DoSatur=off
  Saturation Dynamic1 : simulink/Discontinuities/Saturation Dynamic  OutMin=[]  OutMax=[]  OutDataTypeStr=Inherit: Same as second input  OutDataType=fixdt(1, 16)  OutScaling=2^-10  DoSatur=off
  Saturation Dynamic2 : simulink/Discontinuities/Saturation Dynamic  OutMin=[]  OutMax=[]  OutDataTypeStr=Inherit: Same as second input  OutDataType=fixdt(1, 16)  OutScaling=2^-10  DoSatur=off
  "Speed limit in negative direction of rotation " : Constant  Value=VFD_n_limit_neg_p1086
  Speed limit in positive direction of rotation : Constant  Value=VFD_n_limit_pos_p1083
  Speed limit setpoint channel : Constant  Value=VFD_n_limit_setp_p1063
  Switch : Switch  Criteria=u2 > Threshold
  Switch1 : Switch  Criteria=u2 > Threshold
  "[r1170] n_ctrl setp sum (Speed setpoint after the RFG)" : Outport  VectorParamsAs1DForOutWhenUnconnected=off
  "[r1084] n_limit pos eff Positive Speed limit (rpm)" : Outport  Port=2  VectorParamsAs1DForOutWhenUnconnected=off
  "[r1087] n_limit neg eff Negative Speed limit (rpm)" : Outport  Port=3  VectorParamsAs1DForOutWhenUnconnected=off
  wires:
  Speed limit setpoint channel/1 -> Saturation Dynamic/1, Gain1/1
  Gain1/1 -> Saturation Dynamic/3
  "[p1070(0)] Main Setpoint"/1 -> Gain5/1
  MinMax1/1 -> "[r1087] n_limit neg eff Negative Speed limit (rpm)"/1, Saturation Dynamic1/3
  Saturation Dynamic/1 -> Saturation Dynamic1/2
  Speed limit in positive direction of rotation/1 -> Saturation Dynamic2/1, MinMax/2, MinMax/1
  "Speed limit in negative direction of rotation "/1 -> Saturation Dynamic2/3, MinMax1/2, MinMax1/3
  Maximum speed3/1 -> Gain2/1, MinMax/3
  MinMax/1 -> "[r1084] n_limit pos eff Positive Speed limit (rpm)"/1, Saturation Dynamic1/1
  Saturation Dynamic2/1 -> Gain3/1, Rate Limiter Dynamic/2, Switch/2
  Mux/1 -> Switch/1
  Maximum speed/1 -> Divide1/1
  Demux/2 -> Gain6/1
  Divide3/1 -> Mux1/1, Mux/2
  "Ramp-function generator ramp-up time scaling "/1 -> Divide/1
  Mux1/1 -> Switch/3
  Switch/1 -> Demux/1
  Divide1/1 -> Mux/1, Mux1/2
  "Ramp-function generator ramp-up time "/1 -> Divide/2
  Divide2/1 -> Divide3/2
  Maximum speed1/1 -> Divide3/1
  Ramp-function generator ramp-down time scaling/1 -> Divide2/1
  Ramp-function generator ramp-down time/1 -> Divide2/2
  Divide/1 -> Divide1/2
  Demux/1 -> Rate Limiter Dynamic/1
  Gain4/1 -> "[r1170] n_ctrl setp sum (Speed setpoint after the RFG)"/1  "Speed setpoint after  the ramp function  generator"
  Rate Limiter Dynamic/1 -> Switch1/1
  Switch1/1 -> Gain4/1
  Gain3/1 -> Switch1/3
  Maximum speed2/1 -> Switch1/2
  Gain5/1 -> Saturation Dynamic/2
  Gain6/1 -> Rate Limiter Dynamic/3
  Saturation Dynamic1/1 -> Saturation Dynamic2/2
  Gain2/1 -> MinMax1/1
